simulink model "notlin2"  (Simulink 7.2)
settings: Solver=ode45  StartTime=0  StopTime=0.2
libraries: simulink x6
settings Model: Creator=Admin  ModifiedByFormat=Alexander  LastModifiedBy=Alexander
settings OptimizationCC: BooleanDataType=off  InitFltsAndDblsToZero=on
settings DebuggingCC: SaveWithParameterizedLinksMsg=none  SignalResolutionControl=TryResolveAllWithWarning  SolverPrmCheckMsg=none  MultiTaskDSMMsg=warning  MultiTaskCondExecSysMsg=none  StrictBusMsg=None
settings HardwareCC: TargetUnknown=on
settings RTWCC: IncludeERTFirstTime=on
settings GRTTargetCC: TargetFcnLib=ansi_tfl_tmw.mat

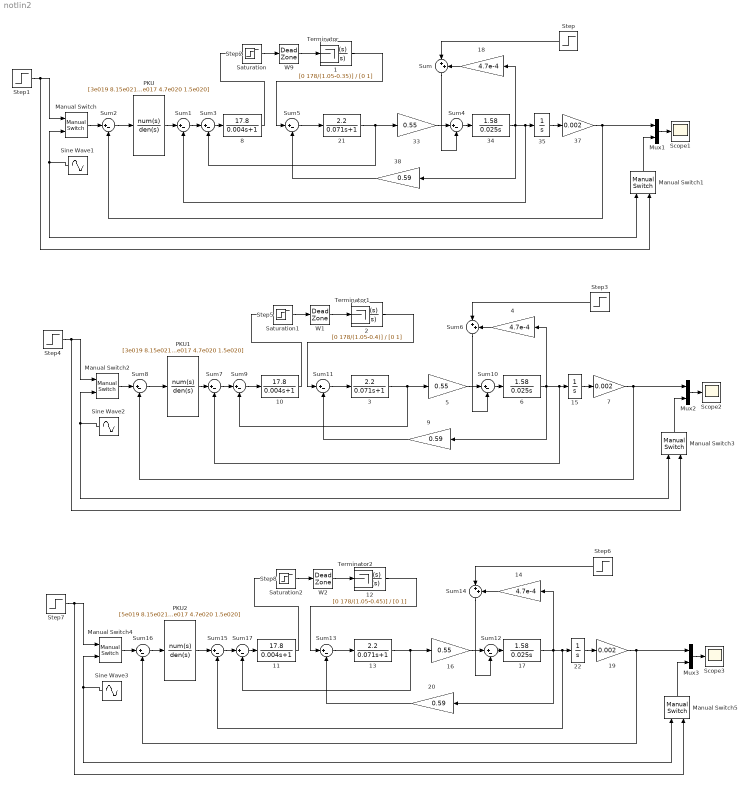
== system notlin2 ==
  1 : TransferFcn  Numerator=[0 178/(1.05-0.35)]  Denominator=[0 1]
  10 : TransferFcn  Numerator=[17.8]  Denominator=[0.004 1]
  11 : TransferFcn  Numerator=[17.8]  Denominator=[0.004 1]
  12 : TransferFcn  Numerator=[0 178/(1.05-0.45)]  Denominator=[0 1]
  13 : TransferFcn  Numerator=[2.2]  Denominator=[0.071 1]
  14 : Gain  Orientation=left  Gain=4.7e-4  ParameterDataType=sfix(16)  ParameterScaling=2^0  OutDataType=sfix(16)  OutScaling=2^0
  15 : TransferFcn  Denominator=[1 0]
  16 : Gain  Gain=0.55  ParameterDataType=sfix(16)  ParameterScaling=2^0  OutDataType=sfix(16)  OutScaling=2^0
  17 : TransferFcn  Numerator=[1.58]  Denominator=[0.025 0]
  18 : Gain  Orientation=left  Gain=4.7e-4  ParameterDataType=sfix(16)  ParameterScaling=2^0  OutDataType=sfix(16)  OutScaling=2^0
  19 : Gain  Gain=0.002  ParameterDataType=sfix(16)  ParameterScaling=2^0  OutDataType=sfix(16)  OutScaling=2^0
  2 : TransferFcn  Numerator=[0 178/(1.05-0.4)]  Denominator=[0 1]
  20 : Gain  Orientation=left  Gain=0.59  ParameterDataType=sfix(16)  ParameterScaling=2^0  OutDataType=sfix(16)  OutScaling=2^0
  21 : TransferFcn  Numerator=[2.2]  Denominator=[0.071 1]
  22 : TransferFcn  Denominator=[1 0]
  3 : TransferFcn  Numerator=[2.2]  Denominator=[0.071 1]
  33 : Gain  Gain=0.55  ParameterDataType=sfix(16)  ParameterScaling=2^0  OutDataType=sfix(16)  OutScaling=2^0
  34 : TransferFcn  Numerator=[1.58]  Denominator=[0.025 0]
  35 : TransferFcn  Denominator=[1 0]
  37 : Gain  Gain=0.002  ParameterDataType=sfix(16)  ParameterScaling=2^0  OutDataType=sfix(16)  OutScaling=2^0
  38 : Gain  Orientation=left  Gain=0.59  ParameterDataType=sfix(16)  ParameterScaling=2^0  OutDataType=sfix(16)  OutScaling=2^0
  4 : Gain  Orientation=left  Gain=4.7e-4  ParameterDataType=sfix(16)  ParameterScaling=2^0  OutDataType=sfix(16)  OutScaling=2^0
  5 : Gain  Gain=0.55  ParameterDataType=sfix(16)  ParameterScaling=2^0  OutDataType=sfix(16)  OutScaling=2^0
  6 : TransferFcn  Numerator=[1.58]  Denominator=[0.025 0]
  7 : Gain  Gain=0.002  ParameterDataType=sfix(16)  ParameterScaling=2^0  OutDataType=sfix(16)  OutScaling=2^0
  8 : TransferFcn  Numerator=[17.8]  Denominator=[0.004 1]
  9 : Gain  Orientation=left  Gain=0.59  ParameterDataType=sfix(16)  ParameterScaling=2^0  OutDataType=sfix(16)  OutScaling=2^0
  Manual Switch : simulink/Signal Routing/Manual Switch  SystemSampleTime=-1  sw=0  action=0  varsize=off
  Manual Switch1 : simulink/Signal Routing/Manual Switch  Orientation=up  SystemSampleTime=-1  sw=1  action=0  varsize=off
  Manual Switch2 : simulink/Signal Routing/Manual Switch  SystemSampleTime=-1  sw=1  action=0  varsize=off
  Manual Switch3 : simulink/Signal Routing/Manual Switch  Orientation=up  SystemSampleTime=-1  sw=0  action=0  varsize=off
  Manual Switch4 : simulink/Signal Routing/Manual Switch  SystemSampleTime=-1  sw=1  action=0  varsize=off
  Manual Switch5 : simulink/Signal Routing/Manual Switch  Orientation=up  SystemSampleTime=-1  sw=0  action=0  varsize=off
  Mux1 : Mux  Inputs=2
  Mux2 : Mux  Inputs=2
  Mux3 : Mux  Inputs=2
  PKU : TransferFcn  Numerator=[3e019 8.15e021 6.4e024 1.5e026 0]  Denominator=[0.059 1.1e004 9.5e008 2e013 1.43e017 4.7e020 1.5e020]
  PKU1 : TransferFcn  Numerator=[3e019 8.15e021 6.4e024 1.5e026 0]  Denominator=[0.059 2.1e004 9.5e008 2e013 1.43e017 4.7e020 1.5e020]
  PKU2 : TransferFcn  Numerator=[5e019 8.15e021 6.4e024 1.5e026 0]  Denominator=[0.059 2.1e004 9.5e008 2e013 1.43e017 4.7e020 1.5e020]
  Saturation : Saturate  UpperLimit=+178  LowerLimit=-178
  Saturation1 : Saturate  UpperLimit=+178  LowerLimit=-178
  Saturation2 : Saturate  UpperLimit=+178  LowerLimit=-178
  Scope1 : Scope
      settings: TickLabels=on  TimeRange=0.2  YMin=-3.5e+020  YMax=4e+020
  Scope2 : Scope
      settings: TickLabels=on  TimeRange=0.1  YMin=0.992  YMax=1
  Scope3 : Scope
      settings: TickLabels=on  TimeRange=0.1  YMin=-0.1  YMax=1.3  SaveName=ScopeData2
  Sine Wave1 : Sin  Orientation=left  Frequency=250  SampleTime=0
  Sine Wave2 : Sin  Orientation=left  Frequency=200  SampleTime=0
  Sine Wave3 : Sin  Orientation=left  Frequency=200  SampleTime=0
  Step : Step  Orientation=left  Time=0  After=1.5  SampleTime=0
  Step1 : Step  Time=0  SampleTime=0
  Step2 : Step  SampleTime=0
  Step3 : Step  Orientation=left  Time=0  After=1.5  SampleTime=0
  Step4 : Step  Time=0  SampleTime=0
  Step5 : Step  SampleTime=0
  Step6 : Step  Orientation=left  Time=0  After=1.5  SampleTime=0
  Step7 : Step  Time=0  SampleTime=0
  Step8 : Step  SampleTime=0
  Sum : Sum  Orientation=down  Inputs=|++  OutDataType=sfix(16)  OutScaling=2^0
  Sum{1..5,7..13,15..17} (15 alike) : Sum  Inputs=|+-  OutDataType=sfix(16)  OutScaling=2^0
  Sum14 : Sum  Orientation=down  Inputs=|++  OutDataType=sfix(16)  OutScaling=2^0
  Sum6 : Sum  Orientation=down  Inputs=|++  OutDataType=sfix(16)  OutScaling=2^0
  Terminator : Terminator
  Terminator1 : Terminator
  Terminator2 : Terminator
  W1 : DeadZone  LowerValue=-0.4  UpperValue=+0.4  SaturateOnIntegerOverflow=on
  W2 : DeadZone  LowerValue=-0.45  UpperValue=+0.45  SaturateOnIntegerOverflow=on
  W9 : DeadZone  LowerValue=-0.35  UpperValue=+0.35  SaturateOnIntegerOverflow=on
  wires:
  Step1/1 -> Manual Switch/1, Manual Switch1/2
  Sine Wave1/1 -> Manual Switch/2, Manual Switch1/1
  Sum5/1 -> 21/1
  21/1 -> 33/1, Sum3/2
  34/1 -> 38/1, Sum1/2, 35/1, 18/1
  38/1 -> Sum5/2
  Mux1/1 -> Scope1/1
  37/1 -> Mux1/1, Sum2/2
  Manual Switch1/1 -> Mux1/2
  Manual Switch/1 -> Sum2/1
  Sum1/1 -> Sum3/1
  Sum3/1 -> 8/1
  Sum2/1 -> PKU/1
  PKU/1 -> Sum1/1
  33/1 -> Sum4/1
  Sum4/1 -> 34/1
  18/1 -> Sum/2
  Step/1 -> Sum/1
  Sum/1 -> Sum4/2
  1/1 -> Terminator/1
  Step2/1 -> Saturation/1
  Saturation/1 -> W9/1
  W9/1 -> 1/1
  8/1 -> Sum5/1
  Step4/1 -> Manual Switch2/1, Manual Switch3/2
  Sine Wave2/1 -> Manual Switch2/2, Manual Switch3/1
  Sum11/1 -> 3/1
  3/1 -> 5/1, Sum9/2
  6/1 -> 9/1, Sum7/2, 15/1, 4/1
  9/1 -> Sum11/2
  Mux2/1 -> Scope2/1
  7/1 -> Mux2/1, Sum8/2
  Manual Switch3/1 -> Mux2/2
  Manual Switch2/1 -> Sum8/1
  Sum7/1 -> Sum9/1
  Sum9/1 -> 10/1
  Sum8/1 -> PKU1/1
  PKU1/1 -> Sum7/1
  5/1 -> Sum10/1
  Sum10/1 -> 6/1
  4/1 -> Sum6/2
  Step3/1 -> Sum6/1
  Sum6/1 -> Sum10/2
  2/1 -> Terminator1/1
  Step5/1 -> Saturation1/1
  Saturation1/1 -> W1/1
  W1/1 -> 2/1
  10/1 -> Sum11/1
  Step7/1 -> Manual Switch4/1, Manual Switch5/2
  Sine Wave3/1 -> Manual Switch4/2, Manual Switch5/1
  Sum13/1 -> 13/1
  13/1 -> 16/1, Sum17/2
  17/1 -> 20/1, Sum15/2, 22/1, 14/1
  20/1 -> Sum13/2
  Mux3/1 -> Scope3/1
  19/1 -> Mux3/1, Sum16/2
  Manual Switch5/1 -> Mux3/2
  Manual Switch4/1 -> Sum16/1
  Sum15/1 -> Sum17/1
  Sum17/1 -> 11/1
  Sum16/1 -> PKU2/1
  PKU2/1 -> Sum15/1
  16/1 -> Sum12/1
  Sum12/1 -> 17/1
  14/1 -> Sum14/2
  Step6/1 -> Sum14/1
  Sum14/1 -> Sum12/2
  12/1 -> Terminator2/1
  Step8/1 -> Saturation2/1
  Saturation2/1 -> W2/1
  W2/1 -> 12/1
  11/1 -> Sum13/1
  15/1 -> 7/1
  22/1 -> 19/1
  35/1 -> 37/1
